simulink model "safebrakingpcont"  (Simulink 7.4)
settings: Solver=ode45  StartTime=0.0  StopTime=40.0  RelTol=1e-3
undefined symbols (not defined in the file): magnitude
settings Model: Creator=Lluís  LastModifiedBy=Lluís
settings SolverCC: ZeroCrossAlgorithm=Adaptive

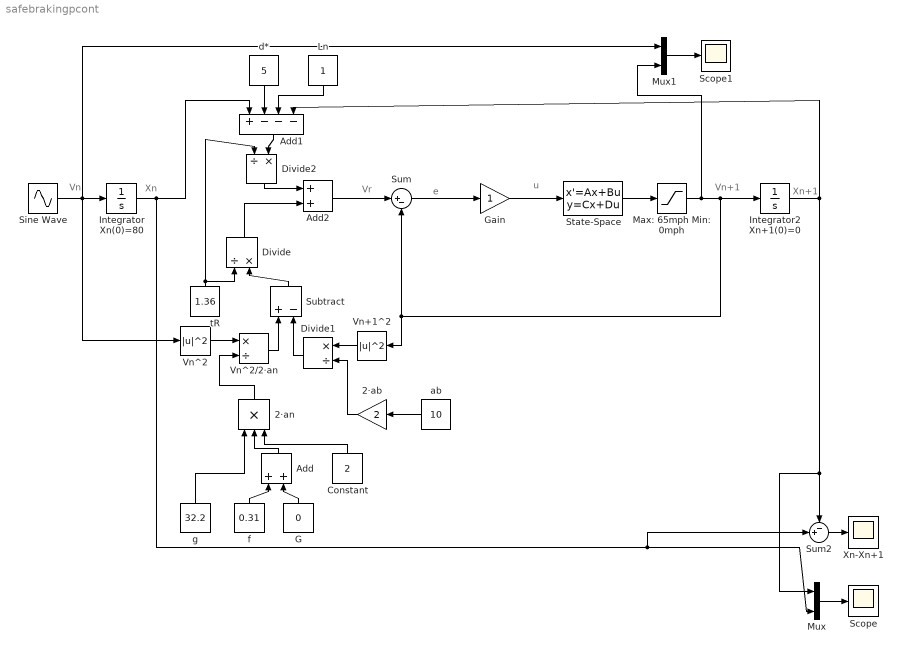
== system safebrakingpcont ==
  note: Vn
  note: Xn
  note: e
  note: u
  note: Vn+1
  note: Xn+1
  note: Vr
  2·ab : Gain  Gain=2  ParameterDataType=fixdt(1, 16)  ParameterScaling=2^0  OutDataType=fixdt(1, 16)  OutScaling=2^0
  2·an : Product  Inputs=3  OutDataType=fixdt(1, 16)  OutScaling=2^0  RndMeth=Zero
  Add : Sum  OutDataType=fixdt(1, 16)  OutScaling=2^-10
  Add1 : Sum  Inputs=+---  OutDataType=fixdt(1, 16)  OutScaling=2^-10
  Add2 : Sum  OutDataType=fixdt(1, 16)  OutScaling=2^-10
  Constant : Constant  Value=2  OutDataType=fixdt(1, 16)  OutScaling=2^0
  Divide : Product  Inputs=/*  OutDataType=fixdt(1, 16)  OutScaling=2^-10
  Divide1 : Product  Inputs=*/  OutDataType=fixdt(1, 16)  OutScaling=2^-10
  Divide2 : Product  Inputs=/*  OutDataType=fixdt(1, 16)  OutScaling=2^-10
  G : Constant  Value=0  OutDataType=fixdt(1, 16)  OutScaling=2^0
  Gain : Gain  ParameterDataType=fixdt(1, 16)  ParameterScaling=2^0  OutDataType=fixdt(1, 16)  OutScaling=2^0
  Integrator Xn(0)=80 : Integrator  InitialCondition=80
  Integrator2 Xn+1(0)=0 : Integrator
  Ln : Constant  OutDataType=fixdt(1, 16)  OutScaling=2^0
  Max: 65mph Min: 0mph : Saturate  UpperLimit=95.33  LowerLimit=0  OutDataType=fixdt(1, 16)  OutScaling=2^0
  Mux : Mux  Inputs=2
  Mux1 : Mux  Inputs=2
  Scope : Scope
  Scope1 : Scope
      settings: SaveName=data2  DataFormat=Array
  Sine Wave : Sin  Amplitude=44  Bias=44  Frequency=2*pi()/10  Phase=0  Samples=10  SampleTime=0  Offset=0
  State-Space : StateSpace  A=0  D=0  X0=44
  Subtract : Sum  Inputs=+-  OutDataType=fixdt(1, 16)  OutScaling=2^-10
  Sum : Sum  Inputs=|+-  OutDataType=fixdt(1, 16)  OutScaling=2^0
  Sum2 : Sum  Inputs=-+|  OutDataType=fixdt(1, 16)  OutScaling=2^0
  Vn+1^2 : Math  Operator=magnitude^2  OutDataType=fixdt(1, 16)  OutScaling=2^0  SaturateOnIntegerOverflow=on
  Vn^2 : Math  Operator=magnitude^2  OutDataType=fixdt(1, 16)  OutScaling=2^0  SaturateOnIntegerOverflow=on
  Vn^2/2·an : Product  Inputs=*/  OutDataType=fixdt(1, 16)  OutScaling=2^-10
  Xn-Xn+1 : Scope
      settings: SaveName=data  DataFormat=Array
  ab : Constant  Value=10  OutDataType=fixdt(1, 16)  OutScaling=2^0
  d* : Constant  Value=5  OutDataType=fixdt(1, 16)  OutScaling=2^0
  f : Constant  Value=0.31  OutDataType=fixdt(1, 16)  OutScaling=2^0
  g : Constant  Value=32.2  OutDataType=fixdt(1, 16)  OutScaling=2^0
  tR : Constant  Value=1.36  OutDataType=fixdt(1, 16)  OutScaling=2^0
  wires:
  Sine Wave/1 -> Integrator Xn(0)=80/1, Vn^2/1, Mux1/1
  State-Space/1 -> Max: 65mph Min: 0mph/1
  Integrator2 Xn+1(0)=0/1 -> Sum2/1, Mux/1, Add1/4
  Max: 65mph Min: 0mph/1 -> Mux1/2, Integrator2 Xn+1(0)=0/1, Sum/2, Vn+1^2/1
  Integrator Xn(0)=80/1 -> Mux/2, Sum2/2, Add1/1
  Add2/1 -> Sum/1
  Sum/1 -> Gain/1
  Gain/1 -> State-Space/1
  f/1 -> Add/1
  G/1 -> Add/2
  Add/1 -> 2·an/2
  g/1 -> 2·an/1
  Constant/1 -> 2·an/3
  ab/1 -> 2·ab/1
  Vn^2/1 -> Vn^2/2·an/1
  2·an/1 -> Vn^2/2·an/2
  Vn+1^2/1 -> Divide1/1
  2·ab/1 -> Divide1/2
  Vn^2/2·an/1 -> Subtract/1
  Divide1/1 -> Subtract/2
  Subtract/1 -> Divide/2
  tR/1 -> Divide/1, Divide2/1
  d*/1 -> Add1/2
  Ln/1 -> Add1/3
  Add1/1 -> Divide2/2
  Divide2/1 -> Add2/1
  Divide/1 -> Add2/2
  Sum2/1 -> Xn-Xn+1/1
  Mux/1 -> Scope/1
  Mux1/1 -> Scope1/1
